simulink model "PID_sim"  (R2018b)
settings: Solver=VariableStepAuto  StartTime=0.0  StopTime=20  RelTol=1e-3
values from neighbouring files (symbols this model uses):
  K_D = 0    [PID_main.m]
  K_I = K_I_vec(i)    [PID_main.m]
  K_P = 1    [PID_main.m]
  RF = rad2deg(0.5)    [PID_main.m]
settings Model: Creator=dhvanipatel  LastModifiedBy=dhvanipatel

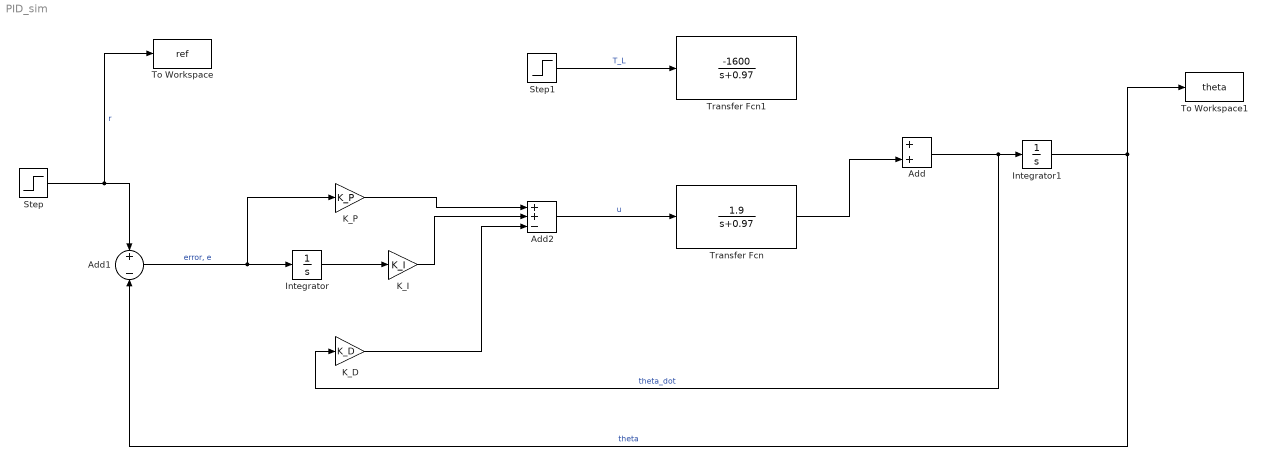
== system PID_sim ==
  Add : Sum
  Add1 : Sum  Inputs=+-
  Add2 : Sum  Inputs=++-
  Integrator : Integrator
  Integrator1 : Integrator
  K_D : Gain  Gain=K_D
  K_I : Gain  Gain=K_I
  K_P : Gain  Gain=K_P
  Step : Step  Time=2  After=RF  SampleTime=0
  Step1 : Step  Time=0  After=0  SampleTime=0
  To Workspace : ToWorkspace  VariableName=ref  SaveFormat=Structure With Time  SampleTime=-1
  To Workspace1 : ToWorkspace  VariableName=theta  SaveFormat=Structure With Time  SampleTime=-1
  Transfer Fcn : TransferFcn  Numerator=1.9  Denominator=[1 0.97]
  Transfer Fcn1 : TransferFcn  Numerator=-1600  Denominator=[1 0.97]
  wires:
  Add2/1 -> Transfer Fcn/1  "u"
  Step1/1 -> Transfer Fcn1/1  "T_L"
  Add/1 -> K_D/1, Integrator1/1  "theta_dot"
  Step/1 -> To Workspace/1, Add1/1  "r"
  Add1/1 -> K_P/1, Integrator/1  "error, e"
  Integrator/1 -> K_I/1
  K_P/1 -> Add2/1
  K_I/1 -> Add2/2
  Integrator1/1 -> Add1/2, To Workspace1/1  "theta"
  Transfer Fcn/1 -> Add/2
  K_D/1 -> Add2/3
